simulink model "fliehkraftpendel"  (Simulink 7.9)
settings: Solver=ode3  StartTime=0.0  StopTime=10.0  FixedStep=1e-3  RelTol=1e-3
values from neighbouring files (symbols this model uses):
  c = 0.05    [Fliehkraftpendel_config.m]
  g = 9.81    [Fliehkraftpendel_config.m]
  l = 0.1    [Fliehkraftpendel_config.m]
  m = 0.5    [Fliehkraftpendel_config.m]
  phi0 = pi/4    (= 0.785398163397)    [Fliehkraftpendel_config.m]
  phipunkt0 = 0    [Fliehkraftpendel_config.m]
  r = 0.01    [Fliehkraftpendel_config.m]
settings Model: Creator=Daniel  LastModifiedBy=Daniel
settings DataIOCC: LimitDataPoints=off

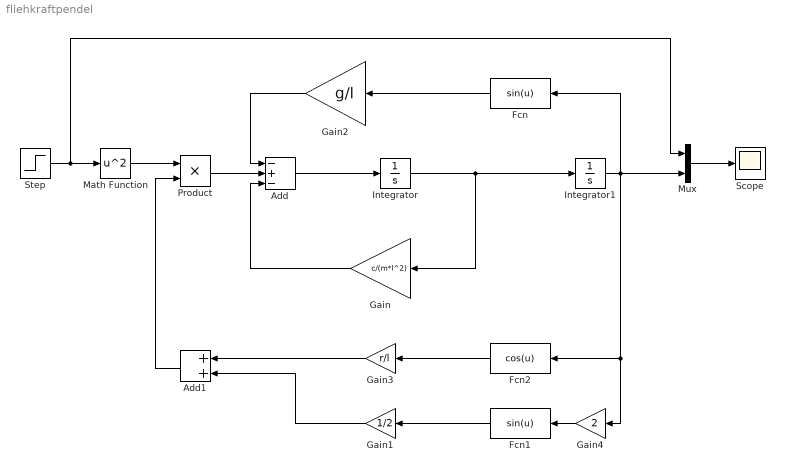
== system fliehkraftpendel ==
  Add : Sum  Inputs=-+-
  Add1 : Sum
  Fcn : Fcn  Expr=sin(u)
  Fcn1 : Fcn  Expr=sin(u)
  Fcn2 : Fcn  Expr=cos(u)
  Gain : Gain  Gain=c/(m*l^2)
  Gain1 : Gain  Gain=1/2
  Gain2 : Gain  Gain=g/l
  Gain3 : Gain  Gain=r/l
  Gain4 : Gain  Gain=2
  Integrator : Integrator  InitialCondition=phipunkt0
  Integrator1 : Integrator  InitialCondition=phi0
  Math Function : Math  Operator=square  SaturateOnIntegerOverflow=on
  Mux : Mux  Inputs=2
  Product : Product  RndMeth=Zero
  Scope : Scope
  Step : Step  Time=4  Before=3  After=12  SampleTime=0
  wires:
  Add/1 -> Integrator/1
  Integrator/1 -> Integrator1/1, Gain/1
  Product/1 -> Add/2
  Integrator1/1 -> Fcn/1, Fcn2/1, Gain4/1, Mux/2
  Fcn/1 -> Gain2/1
  Gain2/1 -> Add/1
  Gain/1 -> Add/3
  Math Function/1 -> Product/1
  Fcn2/1 -> Gain3/1
  Gain3/1 -> Add1/1
  Add1/1 -> Product/2
  Gain4/1 -> Fcn1/1
  Fcn1/1 -> Gain1/1
  Gain1/1 -> Add1/2
  Step/1 -> Math Function/1, Mux/1
  Mux/1 -> Scope/1
